simulink model "DC_Motor"  (R2020a)
settings: Solver=VariableStepAuto  StartTime=0.0  StopTime=10.0  RelTol=1e-3
settings Model: Creator=Souvikdatta  LastModifiedBy=Souvikdatta

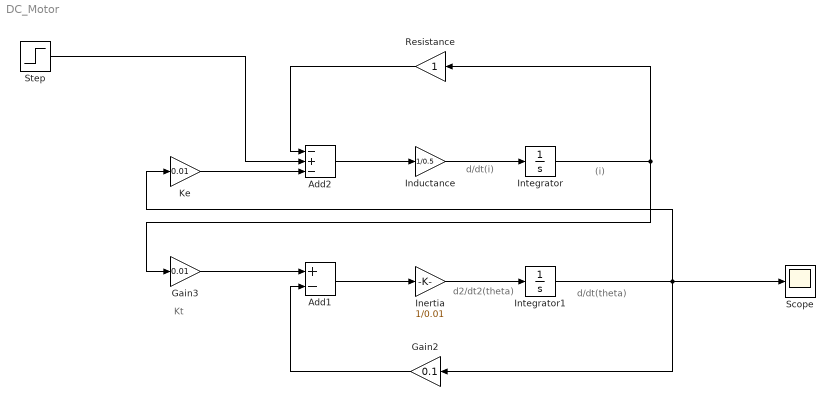
== system DC_Motor ==
  note: d/dt(i)
  note: d2/dt2(theta)
  note: Kt
  note: (i)
  note: d/dt(theta)
  Add1 : Sum  Inputs=+-
  Add2 : Sum  Inputs=-+-
  Gain2 : Gain  Gain=0.1
  Gain3 : Gain  Gain=0.01
  Inductance : Gain  Gain=1/0.5
  Inertia : Gain  Gain=1/0.01
  Integrator : Integrator
  Integrator1 : Integrator
  Ke : Gain  Gain=0.01
  Resistance : Gain
  Scope : Scope
  Step : Step  SampleTime=0
  wires:
  Ke/1 -> Add2/3
  Gain2/1 -> Add1/2
  Integrator/1 -> Resistance/1, Gain3/1
  Inertia/1 -> Integrator1/1
  Inductance/1 -> Integrator/1
  Integrator1/1 -> Scope/1, Ke/1, Gain2/1
  Add1/1 -> Inertia/1
  Gain3/1 -> Add1/1
  Resistance/1 -> Add2/1
  Step/1 -> Add2/2
  Add2/1 -> Inductance/1
